simulink model "Power_System_33Bus_Modeling_test"  (R2024a)
settings: Solver=FixedStepAuto  StartTime=0.0  StopTime=0.2  RelTol=1e-3
libraries: spsThreePhaseSeriesRLCLoadLib x64, spsThreePhaseVIMeasurementLib x33, spsThreePhaseSeriesRLCBranchLib x32, spsRMSLib x2, spsThreePhaseSourceLib x1, spspowerguiLib x1
(part 2 of 2)

== system Power_System_33Bus_Modeling_test/Bus_21 ==
  Bus Load 21 : spsThreePhaseSeriesRLCLoadLib/Three-Phase Series RLC Load  LConnTagsString=A|B|C  Configuration=Y (grounded)  NominalVoltage=22900  Vabc=[1e3 1e3 1e3]  Vabcp=[1e3 1e3 1e3]  NominalFrequency=60  UnbalancedPower=off  ActivePower=450e3  InductivePower=200e3  CapacitivePower=0  Pabc=[10e3 9e3 11e3]  QLabc=[100 90 110]  QCabc=[100 90 110]  Pabcp=[10e3 9e3 11e3]  QLabcp=[100 90 110]  QCabcp=[100 90 110]  Measurements=None  LoadType=constant PQ
  Bus_21 : spsThreePhaseVIMeasurementLib/Three-Phase V-I Measurement  VoltageMeasurement=phase-to-phase  SetLabelV=off  LabelV=Vabc  Vpu=off  VpuLL=off  CurrentMeasurement=yes  SetLabelI=off  LabelI=Iabc  Ipu=off  Pbase=100e6  Vbase=500e3  OutputType=Complex  PhasorSimulation=off  PSBequivalent=0
  Capacitor 21 : spsThreePhaseSeriesRLCLoadLib/Three-Phase Series RLC Load  LConnTagsString=A|B|C  Configuration=Y (grounded)  NominalVoltage=22900  Vabc=[1e3 1e3 1e3]  Vabcp=[1e3 1e3 1e3]  NominalFrequency=60  UnbalancedPower=off  ActivePower=0  InductivePower=0  CapacitivePower=1e-06  Pabc=[10e3 9e3 11e3]  QLabc=[100 90 110]  QCabc=[100 90 110]  Pabcp=[10e3 9e3 11e3]  QLabcp=[100 90 110]  QCabcp=[100 90 110]  Measurements=None  LoadType=constant PQ
  VI Recorder2 : Subsystem
  InPhaseA : PMIOPort  Side=Left
  InPhaseB : PMIOPort  Port=2  Side=Left
  InPhaseC : PMIOPort  Port=3  Side=Left
  OutPhaseA : PMIOPort  Port=4  Side=Right
  OutPhaseB : PMIOPort  Port=5  Side=Right
  OutPhaseC : PMIOPort  Port=6  Side=Right
  wires:
  Bus_21/2 -> VI Recorder2/2(Irec)
  Bus_21/1 -> VI Recorder2/1(Vrec)
  connections:
  Bus Load 21/LConn1 -- Bus_21/RConn1 -- OutPhaseA/RConn1 -- Capacitor 21/LConn1
  Bus Load 21/LConn2 -- Bus_21/RConn2 -- Capacitor 21/LConn2 -- OutPhaseB/RConn1
  Bus_21/RConn3 -- Bus Load 21/LConn3 -- OutPhaseC/RConn1 -- Capacitor 21/LConn3
  InPhaseA/RConn1 -- Bus_21/LConn1
  Bus_21/LConn2 -- InPhaseB/RConn1
  InPhaseC/RConn1 -- Bus_21/LConn3

== system Power_System_33Bus_Modeling_test/Bus_22 ==
  Bus Load 22 : spsThreePhaseSeriesRLCLoadLib/Three-Phase Series RLC Load  LConnTagsString=A|B|C  Configuration=Y (grounded)  NominalVoltage=22900  Vabc=[1e3 1e3 1e3]  Vabcp=[1e3 1e3 1e3]  NominalFrequency=60  UnbalancedPower=off  ActivePower=450e3  InductivePower=200e3  CapacitivePower=0  Pabc=[10e3 9e3 11e3]  QLabc=[100 90 110]  QCabc=[100 90 110]  Pabcp=[10e3 9e3 11e3]  QLabcp=[100 90 110]  QCabcp=[100 90 110]  Measurements=None  LoadType=constant PQ
  Bus_22 : spsThreePhaseVIMeasurementLib/Three-Phase V-I Measurement  VoltageMeasurement=phase-to-phase  SetLabelV=off  LabelV=Vabc  Vpu=off  VpuLL=off  CurrentMeasurement=yes  SetLabelI=off  LabelI=Iabc  Ipu=off  Pbase=100e6  Vbase=500e3  OutputType=Complex  PhasorSimulation=off  PSBequivalent=0
  Capacitor 22 : spsThreePhaseSeriesRLCLoadLib/Three-Phase Series RLC Load  LConnTagsString=A|B|C  Configuration=Y (grounded)  NominalVoltage=22900  Vabc=[1e3 1e3 1e3]  Vabcp=[1e3 1e3 1e3]  NominalFrequency=60  UnbalancedPower=off  ActivePower=0  InductivePower=0  CapacitivePower=1e-06  Pabc=[10e3 9e3 11e3]  QLabc=[100 90 110]  QCabc=[100 90 110]  Pabcp=[10e3 9e3 11e3]  QLabcp=[100 90 110]  QCabcp=[100 90 110]  Measurements=None  LoadType=constant PQ
  VI Recorder3 : Subsystem
  InPhaseA : PMIOPort  Side=Left
  InPhaseB : PMIOPort  Port=2  Side=Left
  InPhaseC : PMIOPort  Port=3  Side=Left
  wires:
  Bus_22/2 -> VI Recorder3/2(Irec)
  Bus_22/1 -> VI Recorder3/1(Vrec)
  connections:
  Bus_22/RConn2 -- Capacitor 22/LConn2 -- Bus Load 22/LConn2
  Bus Load 22/LConn3 -- Capacitor 22/LConn3 -- Bus_22/RConn3
  Bus_22/RConn1 -- Capacitor 22/LConn1 -- Bus Load 22/LConn1
  InPhaseA/RConn1 -- Bus_22/LConn1
  InPhaseB/RConn1 -- Bus_22/LConn2
  InPhaseC/RConn1 -- Bus_22/LConn3

== system Power_System_33Bus_Modeling_test/Bus_23 ==
  Bus Load 23 : spsThreePhaseSeriesRLCLoadLib/Three-Phase Series RLC Load  LConnTagsString=A|B|C  Configuration=Y (grounded)  NominalVoltage=22900  Vabc=[1e3 1e3 1e3]  Vabcp=[1e3 1e3 1e3]  NominalFrequency=60  UnbalancedPower=off  ActivePower=450e3  InductivePower=250e3  CapacitivePower=0  Pabc=[10e3 9e3 11e3]  QLabc=[100 90 110]  QCabc=[100 90 110]  Pabcp=[10e3 9e3 11e3]  QLabcp=[100 90 110]  QCabcp=[100 90 110]  Measurements=None  LoadType=constant PQ
  Bus_23 : spsThreePhaseVIMeasurementLib/Three-Phase V-I Measurement  VoltageMeasurement=phase-to-phase  SetLabelV=off  LabelV=Vabc  Vpu=off  VpuLL=off  CurrentMeasurement=yes  SetLabelI=off  LabelI=Iabc  Ipu=off  Pbase=100e6  Vbase=500e3  OutputType=Complex  PhasorSimulation=off  PSBequivalent=0
  Capacitor 23 : spsThreePhaseSeriesRLCLoadLib/Three-Phase Series RLC Load  LConnTagsString=A|B|C  Configuration=Y (grounded)  NominalVoltage=22900  Vabc=[1e3 1e3 1e3]  Vabcp=[1e3 1e3 1e3]  NominalFrequency=60  UnbalancedPower=off  ActivePower=0  InductivePower=0  CapacitivePower=1e-06  Pabc=[10e3 9e3 11e3]  QLabc=[100 90 110]  QCabc=[100 90 110]  Pabcp=[10e3 9e3 11e3]  QLabcp=[100 90 110]  QCabcp=[100 90 110]  Measurements=None  LoadType=constant PQ
  VI Recorder32 : Subsystem
  InPhaseA : PMIOPort  Side=Left
  InPhaseB : PMIOPort  Port=2  Side=Left
  InPhaseC : PMIOPort  Port=3  Side=Left
  OutPhaseA : PMIOPort  Port=4  Side=Right
  OutPhaseB : PMIOPort  Port=5  Side=Right
  OutPhaseC : PMIOPort  Port=6  Side=Right
  wires:
  Bus_23/2 -> VI Recorder32/2(Irec)
  Bus_23/1 -> VI Recorder32/1(Vrec)
  connections:
  Bus_23/RConn1 -- OutPhaseA/RConn1 -- Capacitor 23/LConn1 -- Bus Load 23/LConn1
  Bus Load 23/LConn2 -- OutPhaseB/RConn1 -- Capacitor 23/LConn2 -- Bus_23/RConn2
  Bus Load 23/LConn3 -- OutPhaseC/RConn1 -- Capacitor 23/LConn3 -- Bus_23/RConn3
  InPhaseA/RConn1 -- Bus_23/LConn1
  InPhaseB/RConn1 -- Bus_23/LConn2
  InPhaseC/RConn1 -- Bus_23/LConn3

== system Power_System_33Bus_Modeling_test/Bus_24 ==
  Bus Load 24 : spsThreePhaseSeriesRLCLoadLib/Three-Phase Series RLC Load  LConnTagsString=A|B|C  Configuration=Y (grounded)  NominalVoltage=22900  Vabc=[1e3 1e3 1e3]  Vabcp=[1e3 1e3 1e3]  NominalFrequency=60  UnbalancedPower=off  ActivePower=2100e3  InductivePower=1000e3  CapacitivePower=0  Pabc=[10e3 9e3 11e3]  QLabc=[100 90 110]  QCabc=[100 90 110]  Pabcp=[10e3 9e3 11e3]  QLabcp=[100 90 110]  QCabcp=[100 90 110]  Measurements=None  LoadType=constant PQ
  Bus_24 : spsThreePhaseVIMeasurementLib/Three-Phase V-I Measurement  VoltageMeasurement=phase-to-phase  SetLabelV=off  LabelV=Vabc  Vpu=off  VpuLL=off  CurrentMeasurement=yes  SetLabelI=off  LabelI=Iabc  Ipu=off  Pbase=100e6  Vbase=500e3  OutputType=Complex  PhasorSimulation=off  PSBequivalent=0
  Capacitor 24 : spsThreePhaseSeriesRLCLoadLib/Three-Phase Series RLC Load  LConnTagsString=A|B|C  Configuration=Y (grounded)  NominalVoltage=22900  Vabc=[1e3 1e3 1e3]  Vabcp=[1e3 1e3 1e3]  NominalFrequency=60  UnbalancedPower=off  ActivePower=0  InductivePower=0  CapacitivePower=1e-06  Pabc=[10e3 9e3 11e3]  QLabc=[100 90 110]  QCabc=[100 90 110]  Pabcp=[10e3 9e3 11e3]  QLabcp=[100 90 110]  QCabcp=[100 90 110]  Measurements=None  LoadType=constant PQ
  VI Recorder31 : Subsystem
  InPhaseA : PMIOPort  Side=Left
  InPhaseB : PMIOPort  Port=2  Side=Left
  InPhaseC : PMIOPort  Port=3  Side=Left
  OutPhaseA : PMIOPort  Port=4  Side=Right
  OutPhaseB : PMIOPort  Port=5  Side=Right
  OutPhaseC : PMIOPort  Port=6  Side=Right
  wires:
  Bus_24/1 -> VI Recorder31/1(Vrec)
  Bus_24/2 -> VI Recorder31/2(Irec)
  connections:
  Bus_24/RConn1 -- OutPhaseA/RConn1 -- Capacitor 24/LConn1 -- Bus Load 24/LConn1
  Bus Load 24/LConn2 -- OutPhaseB/RConn1 -- Capacitor 24/LConn2 -- Bus_24/RConn2
  InPhaseA/RConn1 -- Bus_24/LConn1
  InPhaseB/RConn1 -- Bus_24/LConn2
  InPhaseC/RConn1 -- Bus_24/LConn3
  Bus Load 24/LConn3 -- OutPhaseC/RConn1 -- Capacitor 24/LConn3 -- Bus_24/RConn3

== system Power_System_33Bus_Modeling_test/Bus_25 ==
  Bus Load 25 : spsThreePhaseSeriesRLCLoadLib/Three-Phase Series RLC Load  LConnTagsString=A|B|C  Configuration=Y (grounded)  NominalVoltage=22900  Vabc=[1e3 1e3 1e3]  Vabcp=[1e3 1e3 1e3]  NominalFrequency=60  UnbalancedPower=off  ActivePower=2100e3  InductivePower=1000e3  CapacitivePower=0  Pabc=[10e3 9e3 11e3]  QLabc=[100 90 110]  QCabc=[100 90 110]  Pabcp=[10e3 9e3 11e3]  QLabcp=[100 90 110]  QCabcp=[100 90 110]  Measurements=None  LoadType=constant PQ
  Bus_25 : spsThreePhaseVIMeasurementLib/Three-Phase V-I Measurement  VoltageMeasurement=phase-to-phase  SetLabelV=off  LabelV=Vabc  Vpu=off  VpuLL=off  CurrentMeasurement=yes  SetLabelI=off  LabelI=Iabc  Ipu=off  Pbase=100e6  Vbase=500e3  OutputType=Complex  PhasorSimulation=off  PSBequivalent=0
  Capacitor 25 : spsThreePhaseSeriesRLCLoadLib/Three-Phase Series RLC Load  LConnTagsString=A|B|C  Configuration=Y (grounded)  NominalVoltage=22900  Vabc=[1e3 1e3 1e3]  Vabcp=[1e3 1e3 1e3]  NominalFrequency=60  UnbalancedPower=off  ActivePower=0  InductivePower=0  CapacitivePower=1e-06  Pabc=[10e3 9e3 11e3]  QLabc=[100 90 110]  QCabc=[100 90 110]  Pabcp=[10e3 9e3 11e3]  QLabcp=[100 90 110]  QCabcp=[100 90 110]  Measurements=None  LoadType=constant PQ
  VI Recorder30 : Subsystem
  InPhaseA : PMIOPort  Side=Left
  InPhaseB : PMIOPort  Port=2  Side=Left
  InPhaseC : PMIOPort  Port=3  Side=Left
  wires:
  Bus_25/2 -> VI Recorder30/2(Irec)
  Bus_25/1 -> VI Recorder30/1(Vrec)
  connections:
  Bus Load 25/LConn1 -- Capacitor 25/LConn1 -- Bus_25/RConn1
  Bus_25/RConn2 -- Capacitor 25/LConn2 -- Bus Load 25/LConn2
  Bus Load 25/LConn3 -- Capacitor 25/LConn3 -- Bus_25/RConn3
  InPhaseB/RConn1 -- Bus_25/LConn2
  InPhaseA/RConn1 -- Bus_25/LConn1
  InPhaseC/RConn1 -- Bus_25/LConn3

== system Power_System_33Bus_Modeling_test/Bus_26 ==
  Bus Load 26 : spsThreePhaseSeriesRLCLoadLib/Three-Phase Series RLC Load  LConnTagsString=A|B|C  Configuration=Y (grounded)  NominalVoltage=22900  Vabc=[1e3 1e3 1e3]  Vabcp=[1e3 1e3 1e3]  NominalFrequency=60  UnbalancedPower=off  ActivePower=300e3  InductivePower=125e3  CapacitivePower=0  Pabc=[10e3 9e3 11e3]  QLabc=[100 90 110]  QCabc=[100 90 110]  Pabcp=[10e3 9e3 11e3]  QLabcp=[100 90 110]  QCabcp=[100 90 110]  Measurements=None  LoadType=constant PQ
  Bus_26 : spsThreePhaseVIMeasurementLib/Three-Phase V-I Measurement  VoltageMeasurement=phase-to-phase  SetLabelV=off  LabelV=Vabc  Vpu=off  VpuLL=off  CurrentMeasurement=yes  SetLabelI=off  LabelI=Iabc  Ipu=off  Pbase=100e6  Vbase=500e3  OutputType=Complex  PhasorSimulation=off  PSBequivalent=0
  Capacitor 26 : spsThreePhaseSeriesRLCLoadLib/Three-Phase Series RLC Load  LConnTagsString=A|B|C  Configuration=Y (grounded)  NominalVoltage=22900  Vabc=[1e3 1e3 1e3]  Vabcp=[1e3 1e3 1e3]  NominalFrequency=60  UnbalancedPower=off  ActivePower=0  InductivePower=0  CapacitivePower=1e-06  Pabc=[10e3 9e3 11e3]  QLabc=[100 90 110]  QCabc=[100 90 110]  Pabcp=[10e3 9e3 11e3]  QLabcp=[100 90 110]  QCabcp=[100 90 110]  Measurements=None  LoadType=constant PQ
  VI Recorder22 : Subsystem
  InPhaseA : PMIOPort  Side=Left
  InPhaseB : PMIOPort  Port=2  Side=Left
  InPhaseC : PMIOPort  Port=3  Side=Left
  OutPhaseA : PMIOPort  Port=4  Side=Right
  OutPhaseB : PMIOPort  Port=5  Side=Right
  OutPhaseC : PMIOPort  Port=6  Side=Right
  wires:
  Bus_26/2 -> VI Recorder22/2(Irec)
  Bus_26/1 -> VI Recorder22/1(Vrec)
  connections:
  Bus_26/RConn3 -- OutPhaseC/RConn1 -- Capacitor 26/LConn3 -- Bus Load 26/LConn3
  Bus Load 26/LConn2 -- OutPhaseB/RConn1 -- Capacitor 26/LConn2 -- Bus_26/RConn2
  Bus_26/RConn1 -- OutPhaseA/RConn1 -- Capacitor 26/LConn1 -- Bus Load 26/LConn1
  InPhaseA/RConn1 -- Bus_26/LConn1
  InPhaseB/RConn1 -- Bus_26/LConn2
  InPhaseC/RConn1 -- Bus_26/LConn3

== system Power_System_33Bus_Modeling_test/Bus_27 ==
  Bus Load 27 : spsThreePhaseSeriesRLCLoadLib/Three-Phase Series RLC Load  LConnTagsString=A|B|C  Configuration=Y (grounded)  NominalVoltage=22900  Vabc=[1e3 1e3 1e3]  Vabcp=[1e3 1e3 1e3]  NominalFrequency=60  UnbalancedPower=off  ActivePower=300e3  InductivePower=125e3  CapacitivePower=0  Pabc=[10e3 9e3 11e3]  QLabc=[100 90 110]  QCabc=[100 90 110]  Pabcp=[10e3 9e3 11e3]  QLabcp=[100 90 110]  QCabcp=[100 90 110]  Measurements=None  LoadType=constant PQ
  Bus_27 : spsThreePhaseVIMeasurementLib/Three-Phase V-I Measurement  VoltageMeasurement=phase-to-phase  SetLabelV=off  LabelV=Vabc  Vpu=off  VpuLL=off  CurrentMeasurement=yes  SetLabelI=off  LabelI=Iabc  Ipu=off  Pbase=100e6  Vbase=500e3  OutputType=Complex  PhasorSimulation=off  PSBequivalent=0
  Capacitor 27 : spsThreePhaseSeriesRLCLoadLib/Three-Phase Series RLC Load  LConnTagsString=A|B|C  Configuration=Y (grounded)  NominalVoltage=22900  Vabc=[1e3 1e3 1e3]  Vabcp=[1e3 1e3 1e3]  NominalFrequency=60  UnbalancedPower=off  ActivePower=0  InductivePower=0  CapacitivePower=1e-06  Pabc=[10e3 9e3 11e3]  QLabc=[100 90 110]  QCabc=[100 90 110]  Pabcp=[10e3 9e3 11e3]  QLabcp=[100 90 110]  QCabcp=[100 90 110]  Measurements=None  LoadType=constant PQ
  VI Recorder23 : Subsystem
  InPhaseA : PMIOPort  Side=Left
  InPhaseB : PMIOPort  Port=2  Side=Left
  InPhaseC : PMIOPort  Port=3  Side=Left
  OutPhaseA : PMIOPort  Port=4  Side=Right
  OutPhaseB : PMIOPort  Port=5  Side=Right
  OutPhaseC : PMIOPort  Port=6  Side=Right
  wires:
  Bus_27/1 -> VI Recorder23/1(Vrec)
  Bus_27/2 -> VI Recorder23/2(Irec)
  connections:
  Bus Load 27/LConn1 -- Bus_27/RConn1 -- OutPhaseA/RConn1 -- Capacitor 27/LConn1
  Bus Load 27/LConn2 -- Bus_27/RConn2 -- OutPhaseB/RConn1 -- Capacitor 27/LConn2
  Bus_27/RConn3 -- OutPhaseC/RConn1 -- Capacitor 27/LConn3 -- Bus Load 27/LConn3
  InPhaseA/RConn1 -- Bus_27/LConn1
  InPhaseB/RConn1 -- Bus_27/LConn2
  InPhaseC/RConn1 -- Bus_27/LConn3

== system Power_System_33Bus_Modeling_test/Bus_28 ==
  Bus Load 28 : spsThreePhaseSeriesRLCLoadLib/Three-Phase Series RLC Load  LConnTagsString=A|B|C  Configuration=Y (grounded)  NominalVoltage=22900  Vabc=[1e3 1e3 1e3]  Vabcp=[1e3 1e3 1e3]  NominalFrequency=60  UnbalancedPower=off  ActivePower=300e3  InductivePower=100e3  CapacitivePower=0  Pabc=[10e3 9e3 11e3]  QLabc=[100 90 110]  QCabc=[100 90 110]  Pabcp=[10e3 9e3 11e3]  QLabcp=[100 90 110]  QCabcp=[100 90 110]  Measurements=None  LoadType=constant PQ
  Bus_28 : spsThreePhaseVIMeasurementLib/Three-Phase V-I Measurement  VoltageMeasurement=phase-to-phase  SetLabelV=off  LabelV=Vabc  Vpu=off  VpuLL=off  CurrentMeasurement=yes  SetLabelI=off  LabelI=Iabc  Ipu=off  Pbase=100e6  Vbase=500e3  OutputType=Complex  PhasorSimulation=off  PSBequivalent=0
  Capacitor 28 : spsThreePhaseSeriesRLCLoadLib/Three-Phase Series RLC Load  LConnTagsString=A|B|C  Configuration=Y (grounded)  NominalVoltage=22900  Vabc=[1e3 1e3 1e3]  Vabcp=[1e3 1e3 1e3]  NominalFrequency=60  UnbalancedPower=off  ActivePower=0  InductivePower=0  CapacitivePower=1e-06  Pabc=[10e3 9e3 11e3]  QLabc=[100 90 110]  QCabc=[100 90 110]  Pabcp=[10e3 9e3 11e3]  QLabcp=[100 90 110]  QCabcp=[100 90 110]  Measurements=None  LoadType=constant PQ
  VI Recorder24 : Subsystem
  InPhaseA : PMIOPort  Side=Left
  InPhaseB : PMIOPort  Port=2  Side=Left
  InPhaseC : PMIOPort  Port=3  Side=Left
  OutPhaseA : PMIOPort  Port=4  Side=Right
  OutPhaseB : PMIOPort  Port=5  Side=Right
  OutPhaseC : PMIOPort  Port=6  Side=Right
  wires:
  Bus_28/2 -> VI Recorder24/2(Irec)
  Bus_28/1 -> VI Recorder24/1(Vrec)
  connections:
  Bus Load 28/LConn1 -- OutPhaseA/RConn1 -- Capacitor 28/LConn1 -- Bus_28/RConn1
  Bus Load 28/LConn2 -- OutPhaseB/RConn1 -- Capacitor 28/LConn2 -- Bus_28/RConn2
  Bus Load 28/LConn3 -- OutPhaseC/RConn1 -- Capacitor 28/LConn3 -- Bus_28/RConn3
  InPhaseA/RConn1 -- Bus_28/LConn1
  InPhaseB/RConn1 -- Bus_28/LConn2
  InPhaseC/RConn1 -- Bus_28/LConn3

== system Power_System_33Bus_Modeling_test/Bus_29 ==
  Bus Load 29 : spsThreePhaseSeriesRLCLoadLib/Three-Phase Series RLC Load  LConnTagsString=A|B|C  Configuration=Y (grounded)  NominalVoltage=22900  Vabc=[1e3 1e3 1e3]  Vabcp=[1e3 1e3 1e3]  NominalFrequency=60  UnbalancedPower=off  ActivePower=600e3  InductivePower=350e3  CapacitivePower=0  Pabc=[10e3 9e3 11e3]  QLabc=[100 90 110]  QCabc=[100 90 110]  Pabcp=[10e3 9e3 11e3]  QLabcp=[100 90 110]  QCabcp=[100 90 110]  Measurements=None  LoadType=constant PQ
  Bus_29 : spsThreePhaseVIMeasurementLib/Three-Phase V-I Measurement  VoltageMeasurement=phase-to-phase  SetLabelV=off  LabelV=Vabc  Vpu=off  VpuLL=off  CurrentMeasurement=yes  SetLabelI=off  LabelI=Iabc  Ipu=off  Pbase=100e6  Vbase=500e3  OutputType=Complex  PhasorSimulation=off  PSBequivalent=0
  Capacitor 29 : spsThreePhaseSeriesRLCLoadLib/Three-Phase Series RLC Load  LConnTagsString=A|B|C  Configuration=Y (grounded)  NominalVoltage=22900  Vabc=[1e3 1e3 1e3]  Vabcp=[1e3 1e3 1e3]  NominalFrequency=60  UnbalancedPower=off  ActivePower=0  InductivePower=0  CapacitivePower=1e-06  Pabc=[10e3 9e3 11e3]  QLabc=[100 90 110]  QCabc=[100 90 110]  Pabcp=[10e3 9e3 11e3]  QLabcp=[100 90 110]  QCabcp=[100 90 110]  Measurements=None  LoadType=constant PQ
  VI Recorder25 : Subsystem
  InPhaseA : PMIOPort  Side=Left
  InPhaseB : PMIOPort  Port=2  Side=Left
  InPhaseC : PMIOPort  Port=3  Side=Left
  OutPhaseA : PMIOPort  Port=4  Side=Right
  OutPhaseB : PMIOPort  Port=5  Side=Right
  OutPhaseC : PMIOPort  Port=6  Side=Right
  wires:
  Bus_29/1 -> VI Recorder25/1(Vrec)
  Bus_29/2 -> VI Recorder25/2(Irec)
  connections:
  Bus_29/RConn1 -- OutPhaseA/RConn1 -- Capacitor 29/LConn1 -- Bus Load 29/LConn1
  Bus Load 29/LConn2 -- OutPhaseB/RConn1 -- Capacitor 29/LConn2 -- Bus_29/RConn2
  Bus Load 29/LConn3 -- OutPhaseC/RConn1 -- Capacitor 29/LConn3 -- Bus_29/RConn3
  InPhaseB/RConn1 -- Bus_29/LConn2
  InPhaseA/RConn1 -- Bus_29/LConn1
  InPhaseC/RConn1 -- Bus_29/LConn3

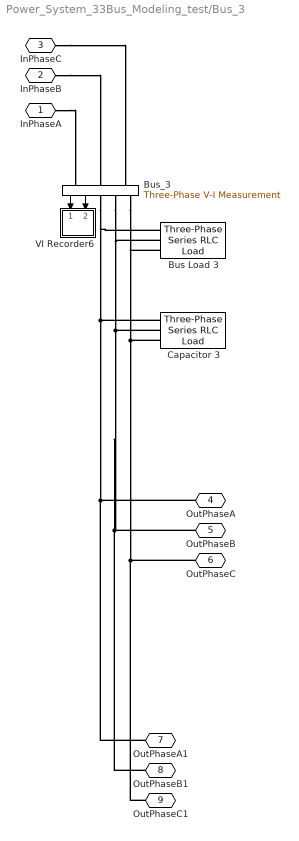
== system Power_System_33Bus_Modeling_test/Bus_3 ==
  Bus Load 3 : spsThreePhaseSeriesRLCLoadLib/Three-Phase Series RLC Load  LConnTagsString=A|B|C  Configuration=Y (grounded)  NominalVoltage=22900  Vabc=[1e3 1e3 1e3]  Vabcp=[1e3 1e3 1e3]  NominalFrequency=60  UnbalancedPower=off  ActivePower=450e3  InductivePower=200e3  CapacitivePower=0  Pabc=[10e3 9e3 11e3]  QLabc=[100 90 110]  QCabc=[100 90 110]  Pabcp=[10e3 9e3 11e3]  QLabcp=[100 90 110]  QCabcp=[100 90 110]  Measurements=None  LoadType=constant PQ
  Bus_3 : spsThreePhaseVIMeasurementLib/Three-Phase V-I Measurement  VoltageMeasurement=phase-to-phase  SetLabelV=off  LabelV=Vabc  Vpu=off  VpuLL=off  CurrentMeasurement=yes  SetLabelI=off  LabelI=Iabc  Ipu=off  Pbase=100e6  Vbase=500e3  OutputType=Complex  PhasorSimulation=off  PSBequivalent=0
  Capacitor 3 : spsThreePhaseSeriesRLCLoadLib/Three-Phase Series RLC Load  LConnTagsString=A|B|C  Configuration=Y (grounded)  NominalVoltage=22900  Vabc=[1e3 1e3 1e3]  Vabcp=[1e3 1e3 1e3]  NominalFrequency=60  UnbalancedPower=off  ActivePower=0  InductivePower=0  CapacitivePower=1e-06  Pabc=[10e3 9e3 11e3]  QLabc=[100 90 110]  QCabc=[100 90 110]  Pabcp=[10e3 9e3 11e3]  QLabcp=[100 90 110]  QCabcp=[100 90 110]  Measurements=None  LoadType=constant PQ
  VI Recorder6 : Subsystem
  InPhaseA : PMIOPort  Side=Left
  InPhaseB : PMIOPort  Port=2  Side=Left
  InPhaseC : PMIOPort  Port=3  Side=Left
  OutPhaseA : PMIOPort  Port=4  Side=Right
  OutPhaseB : PMIOPort  Port=5  Side=Right
  OutPhaseC : PMIOPort  Port=6  Side=Right
  OutPhaseA1 : PMIOPort  Port=7  Side=Right
  OutPhaseB1 : PMIOPort  Port=8  Side=Right
  OutPhaseC1 : PMIOPort  Port=9  Side=Right
  wires:
  Bus_3/2 -> VI Recorder6/2(Irec)
  Bus_3/1 -> VI Recorder6/1(Vrec)
  connections:
  Capacitor 3/LConn1 -- Bus Load 3/LConn1 -- Bus_3/RConn1 -- OutPhaseA1/RConn1 -- OutPhaseA/RConn1
  Capacitor 3/LConn2 -- Bus Load 3/LConn2 -- Bus_3/RConn2 -- OutPhaseB1/RConn1 -- OutPhaseB/RConn1
  Capacitor 3/LConn3 -- Bus_3/RConn3 -- Bus Load 3/LConn3 -- OutPhaseC1/RConn1 -- OutPhaseC/RConn1
  InPhaseA/RConn1 -- Bus_3/LConn1
  InPhaseB/RConn1 -- Bus_3/LConn2
  InPhaseC/RConn1 -- Bus_3/LConn3

== system Power_System_33Bus_Modeling_test/Bus_30 ==
  Bus Load 30 : spsThreePhaseSeriesRLCLoadLib/Three-Phase Series RLC Load  LConnTagsString=A|B|C  Configuration=Y (grounded)  NominalVoltage=22900  Vabc=[1e3 1e3 1e3]  Vabcp=[1e3 1e3 1e3]  NominalFrequency=60  UnbalancedPower=off  ActivePower=1000e3  InductivePower=3000e3  CapacitivePower=0  Pabc=[10e3 9e3 11e3]  QLabc=[100 90 110]  QCabc=[100 90 110]  Pabcp=[10e3 9e3 11e3]  QLabcp=[100 90 110]  QCabcp=[100 90 110]  Measurements=None  LoadType=constant PQ
  Bus_30 : spsThreePhaseVIMeasurementLib/Three-Phase V-I Measurement  VoltageMeasurement=phase-to-phase  SetLabelV=off  LabelV=Vabc  Vpu=off  VpuLL=off  CurrentMeasurement=yes  SetLabelI=off  LabelI=Iabc  Ipu=off  Pbase=100e6  Vbase=500e3  OutputType=Complex  PhasorSimulation=off  PSBequivalent=0
  Capacitor 30 : spsThreePhaseSeriesRLCLoadLib/Three-Phase Series RLC Load  LConnTagsString=A|B|C  Configuration=Y (grounded)  NominalVoltage=22900  Vabc=[1e3 1e3 1e3]  Vabcp=[1e3 1e3 1e3]  NominalFrequency=60  UnbalancedPower=off  ActivePower=0  InductivePower=0  CapacitivePower=1e-06  Pabc=[10e3 9e3 11e3]  QLabc=[100 90 110]  QCabc=[100 90 110]  Pabcp=[10e3 9e3 11e3]  QLabcp=[100 90 110]  QCabcp=[100 90 110]  Measurements=None  LoadType=constant PQ
  VI Recorder26 : Subsystem
  InPhaseA : PMIOPort  Side=Left
  InPhaseB : PMIOPort  Port=2  Side=Left
  InPhaseC : PMIOPort  Port=3  Side=Left
  OutPhaseA : PMIOPort  Port=4  Side=Right
  OutPhaseB : PMIOPort  Port=5  Side=Right
  OutPhaseC : PMIOPort  Port=6  Side=Right
  wires:
  Bus_30/1 -> VI Recorder26/1(Vrec)
  Bus_30/2 -> VI Recorder26/2(Irec)
  connections:
  Bus_30/RConn1 -- OutPhaseA/RConn1 -- Capacitor 30/LConn1 -- Bus Load 30/LConn1
  Bus Load 30/LConn2 -- OutPhaseB/RConn1 -- Capacitor 30/LConn2 -- Bus_30/RConn2
  Bus Load 30/LConn3 -- OutPhaseC/RConn1 -- Capacitor 30/LConn3 -- Bus_30/RConn3
  InPhaseB/RConn1 -- Bus_30/LConn2
  InPhaseA/RConn1 -- Bus_30/LConn1
  InPhaseC/RConn1 -- Bus_30/LConn3

== system Power_System_33Bus_Modeling_test/Bus_31 ==
  Bus Load 31 : spsThreePhaseSeriesRLCLoadLib/Three-Phase Series RLC Load  LConnTagsString=A|B|C  Configuration=Y (grounded)  NominalVoltage=22900  Vabc=[1e3 1e3 1e3]  Vabcp=[1e3 1e3 1e3]  NominalFrequency=60  UnbalancedPower=off  ActivePower=750e3  InductivePower=350e3  CapacitivePower=0  Pabc=[10e3 9e3 11e3]  QLabc=[100 90 110]  QCabc=[100 90 110]  Pabcp=[10e3 9e3 11e3]  QLabcp=[100 90 110]  QCabcp=[100 90 110]  Measurements=None  LoadType=constant PQ
  Bus_31 : spsThreePhaseVIMeasurementLib/Three-Phase V-I Measurement  VoltageMeasurement=phase-to-phase  SetLabelV=off  LabelV=Vabc  Vpu=off  VpuLL=off  CurrentMeasurement=yes  SetLabelI=off  LabelI=Iabc  Ipu=off  Pbase=100e6  Vbase=500e3  OutputType=Complex  PhasorSimulation=off  PSBequivalent=0
  Capacitor 31 : spsThreePhaseSeriesRLCLoadLib/Three-Phase Series RLC Load  LConnTagsString=A|B|C  Configuration=Y (grounded)  NominalVoltage=22900  Vabc=[1e3 1e3 1e3]  Vabcp=[1e3 1e3 1e3]  NominalFrequency=60  UnbalancedPower=off  ActivePower=0  InductivePower=0  CapacitivePower=1e-06  Pabc=[10e3 9e3 11e3]  QLabc=[100 90 110]  QCabc=[100 90 110]  Pabcp=[10e3 9e3 11e3]  QLabcp=[100 90 110]  QCabcp=[100 90 110]  Measurements=None  LoadType=constant PQ
  VI Recorder27 : Subsystem
  InPhaseA : PMIOPort  Side=Left
  InPhaseB : PMIOPort  Port=2  Side=Left
  InPhaseC : PMIOPort  Port=3  Side=Left
  OutPhaseA : PMIOPort  Port=4  Side=Right
  OutPhaseB : PMIOPort  Port=5  Side=Right
  OutPhaseC : PMIOPort  Port=6  Side=Right
  wires:
  Bus_31/2 -> VI Recorder27/2(Irec)
  Bus_31/1 -> VI Recorder27/1(Vrec)
  connections:
  Bus_31/RConn1 -- OutPhaseA/RConn1 -- Capacitor 31/LConn1 -- Bus Load 31/LConn1
  Bus Load 31/LConn2 -- OutPhaseB/RConn1 -- Capacitor 31/LConn2 -- Bus_31/RConn2
  Bus Load 31/LConn3 -- OutPhaseC/RConn1 -- Capacitor 31/LConn3 -- Bus_31/RConn3
  InPhaseA/RConn1 -- Bus_31/LConn1
  Bus_31/LConn2 -- InPhaseB/RConn1
  InPhaseC/RConn1 -- Bus_31/LConn3

== system Power_System_33Bus_Modeling_test/Bus_32 ==
  Bus Load 32 : spsThreePhaseSeriesRLCLoadLib/Three-Phase Series RLC Load  LConnTagsString=A|B|C  Configuration=Y (grounded)  NominalVoltage=22900  Vabc=[1e3 1e3 1e3]  Vabcp=[1e3 1e3 1e3]  NominalFrequency=60  UnbalancedPower=off  ActivePower=1050e3  InductivePower=500e3  CapacitivePower=0  Pabc=[10e3 9e3 11e3]  QLabc=[100 90 110]  QCabc=[100 90 110]  Pabcp=[10e3 9e3 11e3]  QLabcp=[100 90 110]  QCabcp=[100 90 110]  Measurements=None  LoadType=constant PQ
  Bus_32 : spsThreePhaseVIMeasurementLib/Three-Phase V-I Measurement  VoltageMeasurement=phase-to-phase  SetLabelV=off  LabelV=Vabc  Vpu=off  VpuLL=off  CurrentMeasurement=yes  SetLabelI=off  LabelI=Iabc  Ipu=off  Pbase=100e6  Vbase=500e3  OutputType=Complex  PhasorSimulation=off  PSBequivalent=0
  Capacitor 32 : spsThreePhaseSeriesRLCLoadLib/Three-Phase Series RLC Load  LConnTagsString=A|B|C  Configuration=Y (grounded)  NominalVoltage=22900  Vabc=[1e3 1e3 1e3]  Vabcp=[1e3 1e3 1e3]  NominalFrequency=60  UnbalancedPower=off  ActivePower=0  InductivePower=0  CapacitivePower=1e-06  Pabc=[10e3 9e3 11e3]  QLabc=[100 90 110]  QCabc=[100 90 110]  Pabcp=[10e3 9e3 11e3]  QLabcp=[100 90 110]  QCabcp=[100 90 110]  Measurements=None  LoadType=constant PQ
  VI Recorder28 : Subsystem
  InPhaseA : PMIOPort  Side=Left
  InPhaseB : PMIOPort  Port=2  Side=Left
  InPhaseC : PMIOPort  Port=3  Side=Left
  OutPhaseA : PMIOPort  Port=4  Side=Right
  OutPhaseB : PMIOPort  Port=5  Side=Right
  OutPhaseC : PMIOPort  Port=6  Side=Right
  wires:
  Bus_32/2 -> VI Recorder28/2(Irec)
  Bus_32/1 -> VI Recorder28/1(Vrec)
  connections:
  Bus_32/RConn1 -- OutPhaseA/RConn1 -- Capacitor 32/LConn1 -- Bus Load 32/LConn1
  Bus_32/RConn3 -- OutPhaseC/RConn1 -- Capacitor 32/LConn3 -- Bus Load 32/LConn3
  Bus Load 32/LConn2 -- OutPhaseB/RConn1 -- Capacitor 32/LConn2 -- Bus_32/RConn2
  InPhaseA/RConn1 -- Bus_32/LConn1
  InPhaseB/RConn1 -- Bus_32/LConn2
  InPhaseC/RConn1 -- Bus_32/LConn3

== system Power_System_33Bus_Modeling_test/Bus_33 ==
  Bus Load 33 : spsThreePhaseSeriesRLCLoadLib/Three-Phase Series RLC Load  LConnTagsString=A|B|C  Configuration=Y (grounded)  NominalVoltage=22900  Vabc=[1e3 1e3 1e3]  Vabcp=[1e3 1e3 1e3]  NominalFrequency=60  UnbalancedPower=off  ActivePower=300e3  InductivePower=200e3  CapacitivePower=0  Pabc=[10e3 9e3 11e3]  QLabc=[100 90 110]  QCabc=[100 90 110]  Pabcp=[10e3 9e3 11e3]  QLabcp=[100 90 110]  QCabcp=[100 90 110]  Measurements=None  LoadType=constant PQ
  Bus_33 : spsThreePhaseVIMeasurementLib/Three-Phase V-I Measurement  VoltageMeasurement=phase-to-phase  SetLabelV=off  LabelV=Vabc  Vpu=off  VpuLL=off  CurrentMeasurement=yes  SetLabelI=off  LabelI=Iabc  Ipu=off  Pbase=100e6  Vbase=500e3  OutputType=Complex  PhasorSimulation=off  PSBequivalent=0
  Capacitor 33 : spsThreePhaseSeriesRLCLoadLib/Three-Phase Series RLC Load  LConnTagsString=A|B|C  Configuration=Y (grounded)  NominalVoltage=22900  Vabc=[1e3 1e3 1e3]  Vabcp=[1e3 1e3 1e3]  NominalFrequency=60  UnbalancedPower=off  ActivePower=0  InductivePower=0  CapacitivePower=1e-06  Pabc=[10e3 9e3 11e3]  QLabc=[100 90 110]  QCabc=[100 90 110]  Pabcp=[10e3 9e3 11e3]  QLabcp=[100 90 110]  QCabcp=[100 90 110]  Measurements=None  LoadType=constant PQ
  VI Recorder29 : Subsystem
  InPhaseA : PMIOPort  Side=Left
  InPhaseB : PMIOPort  Port=2  Side=Left
  InPhaseC : PMIOPort  Port=3  Side=Left
  wires:
  Bus_33/2 -> VI Recorder29/2(Irec)
  Bus_33/1 -> VI Recorder29/1(Vrec)
  connections:
  Bus Load 33/LConn1 -- Capacitor 33/LConn1 -- Bus_33/RConn1
  Bus Load 33/LConn2 -- Capacitor 33/LConn2 -- Bus_33/RConn2
  Bus_33/RConn3 -- Capacitor 33/LConn3 -- Bus Load 33/LConn3
  InPhaseA/RConn1 -- Bus_33/LConn1
  InPhaseB/RConn1 -- Bus_33/LConn2
  InPhaseC/RConn1 -- Bus_33/LConn3

== system Power_System_33Bus_Modeling_test/Bus_4 ==
  Bus Load 4 : spsThreePhaseSeriesRLCLoadLib/Three-Phase Series RLC Load  LConnTagsString=A|B|C  Configuration=Y (grounded)  NominalVoltage=22900  Vabc=[1e3 1e3 1e3]  Vabcp=[1e3 1e3 1e3]  NominalFrequency=60  UnbalancedPower=off  ActivePower=600e3  InductivePower=400e3  CapacitivePower=0  Pabc=[10e3 9e3 11e3]  QLabc=[100 90 110]  QCabc=[100 90 110]  Pabcp=[10e3 9e3 11e3]  QLabcp=[100 90 110]  QCabcp=[100 90 110]  Measurements=None  LoadType=constant PQ
  Bus_4 : spsThreePhaseVIMeasurementLib/Three-Phase V-I Measurement  VoltageMeasurement=phase-to-phase  SetLabelV=off  LabelV=Vabc  Vpu=off  VpuLL=off  CurrentMeasurement=yes  SetLabelI=off  LabelI=Iabc  Ipu=off  Pbase=100e6  Vbase=500e3  OutputType=Complex  PhasorSimulation=off  PSBequivalent=0
  Capacitor 4 : spsThreePhaseSeriesRLCLoadLib/Three-Phase Series RLC Load  LConnTagsString=A|B|C  Configuration=Y (grounded)  NominalVoltage=22900  Vabc=[1e3 1e3 1e3]  Vabcp=[1e3 1e3 1e3]  NominalFrequency=60  UnbalancedPower=off  ActivePower=0  InductivePower=0  CapacitivePower=1e-06  Pabc=[10e3 9e3 11e3]  QLabc=[100 90 110]  QCabc=[100 90 110]  Pabcp=[10e3 9e3 11e3]  QLabcp=[100 90 110]  QCabcp=[100 90 110]  Measurements=None  LoadType=constant PQ
  VI Recorder7 : Subsystem
  InPhaseA : PMIOPort  Side=Left
  InPhaseB : PMIOPort  Port=2  Side=Left
  InPhaseC : PMIOPort  Port=3  Side=Left
  OutPhaseA : PMIOPort  Port=4  Side=Right
  OutPhaseB : PMIOPort  Port=5  Side=Right
  OutPhaseC : PMIOPort  Port=6  Side=Right
  wires:
  Bus_4/1 -> VI Recorder7/1(Vrec)
  Bus_4/2 -> VI Recorder7/2(Irec)
  connections:
  Bus_4/RConn1 -- OutPhaseA/RConn1 -- Capacitor 4/LConn1 -- Bus Load 4/LConn1
  Bus Load 4/LConn2 -- OutPhaseB/RConn1 -- Capacitor 4/LConn2 -- Bus_4/RConn2
  Bus_4/RConn3 -- OutPhaseC/RConn1 -- Capacitor 4/LConn3 -- Bus Load 4/LConn3
  InPhaseA/RConn1 -- Bus_4/LConn1
  InPhaseB/RConn1 -- Bus_4/LConn2
  InPhaseC/RConn1 -- Bus_4/LConn3

== system Power_System_33Bus_Modeling_test/Bus_5 ==
  Bus Load 5 : spsThreePhaseSeriesRLCLoadLib/Three-Phase Series RLC Load  LConnTagsString=A|B|C  Configuration=Y (grounded)  NominalVoltage=22900  Vabc=[1e3 1e3 1e3]  Vabcp=[1e3 1e3 1e3]  NominalFrequency=50  UnbalancedPower=off  ActivePower=300e3  InductivePower=150e3  CapacitivePower=0  Pabc=[10e3 9e3 11e3]  QLabc=[100 90 110]  QCabc=[100 90 110]  Pabcp=[10e3 9e3 11e3]  QLabcp=[100 90 110]  QCabcp=[100 90 110]  Measurements=None  LoadType=constant PQ
  Bus_5 : spsThreePhaseVIMeasurementLib/Three-Phase V-I Measurement  VoltageMeasurement=phase-to-phase  SetLabelV=off  LabelV=Vabc  Vpu=off  VpuLL=off  CurrentMeasurement=yes  SetLabelI=off  LabelI=Iabc  Ipu=off  Pbase=100e6  Vbase=500e3  OutputType=Complex  PhasorSimulation=off  PSBequivalent=0
  Capacitor 5 : spsThreePhaseSeriesRLCLoadLib/Three-Phase Series RLC Load  LConnTagsString=A|B|C  Configuration=Y (grounded)  NominalVoltage=22900  Vabc=[1e3 1e3 1e3]  Vabcp=[1e3 1e3 1e3]  NominalFrequency=60  UnbalancedPower=off  ActivePower=0  InductivePower=0  CapacitivePower=1e-06  Pabc=[10e3 9e3 11e3]  QLabc=[100 90 110]  QCabc=[100 90 110]  Pabcp=[10e3 9e3 11e3]  QLabcp=[100 90 110]  QCabcp=[100 90 110]  Measurements=None  LoadType=constant PQ
  VI Recorder8 : Subsystem
  InPhaseA : PMIOPort  Side=Left
  InPhaseB : PMIOPort  Port=2  Side=Left
  InPhaseC : PMIOPort  Port=3  Side=Left
  OutPhaseA : PMIOPort  Port=4  Side=Right
  OutPhaseB : PMIOPort  Port=5  Side=Right
  OutPhaseC : PMIOPort  Port=6  Side=Right
  wires:
  Bus_5/2 -> VI Recorder8/2(Irec)
  Bus_5/1 -> VI Recorder8/1(Vrec)
  connections:
  Bus Load 5/LConn1 -- OutPhaseA/RConn1 -- Capacitor 5/LConn1 -- Bus_5/RConn1
  Bus_5/RConn2 -- OutPhaseB/RConn1 -- Capacitor 5/LConn2 -- Bus Load 5/LConn2
  Bus_5/RConn3 -- OutPhaseC/RConn1 -- Capacitor 5/LConn3 -- Bus Load 5/LConn3
  InPhaseA/RConn1 -- Bus_5/LConn1
  InPhaseB/RConn1 -- Bus_5/LConn2
  InPhaseC/RConn1 -- Bus_5/LConn3

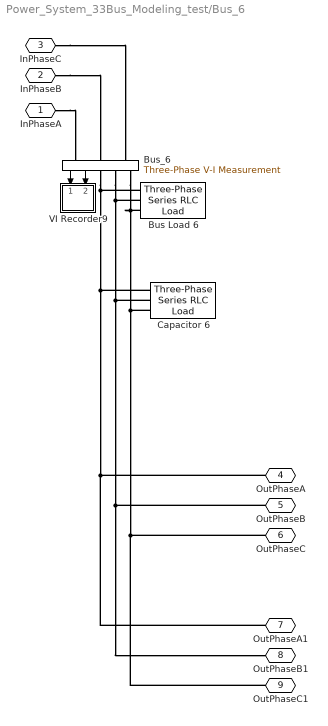
== system Power_System_33Bus_Modeling_test/Bus_6 ==
  Bus Load 6 : spsThreePhaseSeriesRLCLoadLib/Three-Phase Series RLC Load  LConnTagsString=A|B|C  Configuration=Y (grounded)  NominalVoltage=22900  Vabc=[1e3 1e3 1e3]  Vabcp=[1e3 1e3 1e3]  NominalFrequency=60  UnbalancedPower=off  ActivePower=300e3  InductivePower=100e3  CapacitivePower=0  Pabc=[10e3 9e3 11e3]  QLabc=[100 90 110]  QCabc=[100 90 110]  Pabcp=[10e3 9e3 11e3]  QLabcp=[100 90 110]  QCabcp=[100 90 110]  Measurements=None  LoadType=constant PQ
  Bus_6 : spsThreePhaseVIMeasurementLib/Three-Phase V-I Measurement  VoltageMeasurement=phase-to-phase  SetLabelV=off  LabelV=Vabc  Vpu=off  VpuLL=off  CurrentMeasurement=yes  SetLabelI=off  LabelI=Iabc  Ipu=off  Pbase=100e6  Vbase=500e3  OutputType=Complex  PhasorSimulation=off  PSBequivalent=0
  Capacitor 6 : spsThreePhaseSeriesRLCLoadLib/Three-Phase Series RLC Load  LConnTagsString=A|B|C  Configuration=Y (grounded)  NominalVoltage=22900  Vabc=[1e3 1e3 1e3]  Vabcp=[1e3 1e3 1e3]  NominalFrequency=60  UnbalancedPower=off  ActivePower=0  InductivePower=0  CapacitivePower=1e-06  Pabc=[10e3 9e3 11e3]  QLabc=[100 90 110]  QCabc=[100 90 110]  Pabcp=[10e3 9e3 11e3]  QLabcp=[100 90 110]  QCabcp=[100 90 110]  Measurements=None  LoadType=constant PQ
  VI Recorder9 : Subsystem
  InPhaseA : PMIOPort  Side=Left
  InPhaseB : PMIOPort  Port=2  Side=Left
  InPhaseC : PMIOPort  Port=3  Side=Left
  OutPhaseA : PMIOPort  Port=4  Side=Right
  OutPhaseB : PMIOPort  Port=5  Side=Right
  OutPhaseC : PMIOPort  Port=6  Side=Right
  OutPhaseA1 : PMIOPort  Port=7  Side=Right
  OutPhaseB1 : PMIOPort  Port=8  Side=Right
  OutPhaseC1 : PMIOPort  Port=9  Side=Right
  wires:
  Bus_6/1 -> VI Recorder9/1(Vrec)
  Bus_6/2 -> VI Recorder9/2(Irec)
  connections:
  Bus Load 6/LConn1 -- Capacitor 6/LConn1 -- OutPhaseA1/RConn1 -- OutPhaseA/RConn1 -- Bus_6/RConn1
  Bus Load 6/LConn3 -- Capacitor 6/LConn3 -- OutPhaseC1/RConn1 -- OutPhaseC/RConn1 -- Bus_6/RConn3
  Bus Load 6/LConn2 -- Capacitor 6/LConn2 -- OutPhaseB/RConn1 -- OutPhaseB1/RConn1 -- Bus_6/RConn2
  InPhaseA/RConn1 -- Bus_6/LConn1
  InPhaseB/RConn1 -- Bus_6/LConn2
  InPhaseC/RConn1 -- Bus_6/LConn3

== system Power_System_33Bus_Modeling_test/Bus_7 ==
  Bus Load 7 : spsThreePhaseSeriesRLCLoadLib/Three-Phase Series RLC Load  LConnTagsString=A|B|C  Configuration=Y (grounded)  NominalVoltage=22900  Vabc=[1e3 1e3 1e3]  Vabcp=[1e3 1e3 1e3]  NominalFrequency=60  UnbalancedPower=off  ActivePower=1000e3  InductivePower=500e3  CapacitivePower=0  Pabc=[10e3 9e3 11e3]  QLabc=[100 90 110]  QCabc=[100 90 110]  Pabcp=[10e3 9e3 11e3]  QLabcp=[100 90 110]  QCabcp=[100 90 110]  Measurements=None  LoadType=constant PQ
  Bus_7 : spsThreePhaseVIMeasurementLib/Three-Phase V-I Measurement  VoltageMeasurement=phase-to-phase  SetLabelV=off  LabelV=Vabc  Vpu=off  VpuLL=off  CurrentMeasurement=yes  SetLabelI=off  LabelI=Iabc  Ipu=off  Pbase=100e6  Vbase=500e3  OutputType=Complex  PhasorSimulation=off  PSBequivalent=0
  Capacitor 7 : spsThreePhaseSeriesRLCLoadLib/Three-Phase Series RLC Load  LConnTagsString=A|B|C  Configuration=Y (grounded)  NominalVoltage=22900  Vabc=[1e3 1e3 1e3]  Vabcp=[1e3 1e3 1e3]  NominalFrequency=60  UnbalancedPower=off  ActivePower=0  InductivePower=0  CapacitivePower=1e-06  Pabc=[10e3 9e3 11e3]  QLabc=[100 90 110]  QCabc=[100 90 110]  Pabcp=[10e3 9e3 11e3]  QLabcp=[100 90 110]  QCabcp=[100 90 110]  Measurements=None  LoadType=constant PQ
  VI Recorder10 : Subsystem
  InPhaseA : PMIOPort  Side=Left
  InPhaseB : PMIOPort  Port=2  Side=Left
  InPhaseC : PMIOPort  Port=3  Side=Left
  OutPhaseA : PMIOPort  Port=4  Side=Right
  OutPhaseB : PMIOPort  Port=5  Side=Right
  OutPhaseC : PMIOPort  Port=6  Side=Right
  wires:
  Bus_7/2 -> VI Recorder10/2(Irec)
  Bus_7/1 -> VI Recorder10/1(Vrec)
  connections:
  Bus_7/RConn1 -- OutPhaseA/RConn1 -- Capacitor 7/LConn1 -- Bus Load 7/LConn1
  Bus Load 7/LConn2 -- OutPhaseB/RConn1 -- Capacitor 7/LConn2 -- Bus_7/RConn2
  Capacitor 7/LConn3 -- OutPhaseC/RConn1 -- Bus Load 7/LConn3 -- Bus_7/RConn3
  InPhaseA/RConn1 -- Bus_7/LConn1
  InPhaseB/RConn1 -- Bus_7/LConn2
  InPhaseC/RConn1 -- Bus_7/LConn3

== system Power_System_33Bus_Modeling_test/Bus_8 ==
  Bus Load 8 : spsThreePhaseSeriesRLCLoadLib/Three-Phase Series RLC Load  LConnTagsString=A|B|C  Configuration=Y (grounded)  NominalVoltage=22900  Vabc=[1e3 1e3 1e3]  Vabcp=[1e3 1e3 1e3]  NominalFrequency=60  UnbalancedPower=off  ActivePower=1000e3  InductivePower=500e3  CapacitivePower=0  Pabc=[10e3 9e3 11e3]  QLabc=[100 90 110]  QCabc=[100 90 110]  Pabcp=[10e3 9e3 11e3]  QLabcp=[100 90 110]  QCabcp=[100 90 110]  Measurements=None  LoadType=constant PQ
  Bus_8 : spsThreePhaseVIMeasurementLib/Three-Phase V-I Measurement  VoltageMeasurement=phase-to-phase  SetLabelV=off  LabelV=Vabc  Vpu=off  VpuLL=off  CurrentMeasurement=yes  SetLabelI=off  LabelI=Iabc  Ipu=off  Pbase=100e6  Vbase=500e3  OutputType=Complex  PhasorSimulation=off  PSBequivalent=0
  Capacitor 8 : spsThreePhaseSeriesRLCLoadLib/Three-Phase Series RLC Load  LConnTagsString=A|B|C  Configuration=Y (grounded)  NominalVoltage=22900  Vabc=[1e3 1e3 1e3]  Vabcp=[1e3 1e3 1e3]  NominalFrequency=60  UnbalancedPower=off  ActivePower=0  InductivePower=0  CapacitivePower=1e-06  Pabc=[10e3 9e3 11e3]  QLabc=[100 90 110]  QCabc=[100 90 110]  Pabcp=[10e3 9e3 11e3]  QLabcp=[100 90 110]  QCabcp=[100 90 110]  Measurements=None  LoadType=constant PQ
  VI Recorder11 : Subsystem
  OutPhaseA : PMIOPort  Side=Right
  OutPhaseB : PMIOPort  Port=2  Side=Right
  OutPhaseC : PMIOPort  Port=3  Side=Right
  InPhaseA1 : PMIOPort  Port=4  Side=Left
  InPhaseB1 : PMIOPort  Port=5  Side=Left
  InPhaseC1 : PMIOPort  Port=6  Side=Left
  wires:
  Bus_8/2 -> VI Recorder11/2(Irec)
  Bus_8/1 -> VI Recorder11/1(Vrec)
  connections:
  Bus Load 8/LConn1 -- OutPhaseA/RConn1 -- Capacitor 8/LConn1 -- Bus_8/RConn1
  Bus Load 8/LConn2 -- OutPhaseB/RConn1 -- Capacitor 8/LConn2 -- Bus_8/RConn2
  Bus_8/RConn3 -- OutPhaseC/RConn1 -- Capacitor 8/LConn3 -- Bus Load 8/LConn3
  InPhaseA1/RConn1 -- Bus_8/LConn1
  InPhaseB1/RConn1 -- Bus_8/LConn2
  InPhaseC1/RConn1 -- Bus_8/LConn3

== system Power_System_33Bus_Modeling_test/Bus_9 ==
  Bus Load 9 : spsThreePhaseSeriesRLCLoadLib/Three-Phase Series RLC Load  LConnTagsString=A|B|C  Configuration=Y (grounded)  NominalVoltage=22900  Vabc=[1e3 1e3 1e3]  Vabcp=[1e3 1e3 1e3]  NominalFrequency=60  UnbalancedPower=off  ActivePower=300e3  InductivePower=100e3  CapacitivePower=0  Pabc=[10e3 9e3 11e3]  QLabc=[100 90 110]  QCabc=[100 90 110]  Pabcp=[10e3 9e3 11e3]  QLabcp=[100 90 110]  QCabcp=[100 90 110]  Measurements=None  LoadType=constant PQ
  Bus_9 : spsThreePhaseVIMeasurementLib/Three-Phase V-I Measurement  VoltageMeasurement=phase-to-phase  SetLabelV=off  LabelV=Vabc  Vpu=off  VpuLL=off  CurrentMeasurement=yes  SetLabelI=off  LabelI=Iabc  Ipu=off  Pbase=100e6  Vbase=500e3  OutputType=Complex  PhasorSimulation=off  PSBequivalent=0
  Capacitor 9 : spsThreePhaseSeriesRLCLoadLib/Three-Phase Series RLC Load  LConnTagsString=A|B|C  Configuration=Y (grounded)  NominalVoltage=22900  Vabc=[1e3 1e3 1e3]  Vabcp=[1e3 1e3 1e3]  NominalFrequency=60  UnbalancedPower=off  ActivePower=0  InductivePower=0  CapacitivePower=1e-06  Pabc=[10e3 9e3 11e3]  QLabc=[100 90 110]  QCabc=[100 90 110]  Pabcp=[10e3 9e3 11e3]  QLabcp=[100 90 110]  QCabcp=[100 90 110]  Measurements=None  LoadType=constant PQ
  VI Recorder12 : Subsystem
  InPhaseA : PMIOPort  Side=Left
  InPhaseB : PMIOPort  Port=2  Side=Left
  InPhaseC : PMIOPort  Port=3  Side=Left
  OutPhaseA : PMIOPort  Port=4  Side=Right
  OutPhaseB : PMIOPort  Port=5  Side=Right
  OutPhaseC : PMIOPort  Port=6  Side=Right
  wires:
  Bus_9/2 -> VI Recorder12/2(Irec)
  Bus_9/1 -> VI Recorder12/1(Vrec)
  connections:
  Capacitor 9/LConn1 -- OutPhaseA/RConn1 -- Bus Load 9/LConn1 -- Bus_9/RConn1
  Capacitor 9/LConn2 -- OutPhaseB/RConn1 -- Bus_9/RConn2 -- Bus Load 9/LConn2
  Bus Load 9/LConn3 -- Bus_9/RConn3 -- OutPhaseC/RConn1 -- Capacitor 9/LConn3
  InPhaseA/RConn1 -- Bus_9/LConn1
  InPhaseB/RConn1 -- Bus_9/LConn2
  InPhaseC/RConn1 -- Bus_9/LConn3

== system Power_System_33Bus_Modeling_test/Bus_10/VI Recorder13 ==
  Vrec : Inport
  Irec : Inport  Port=2
  tag scope: I9to10=global, V9to10=global
  wires:
  Vrec/1 -> [V9to10]
  Irec/1 -> [I9to10]

== system Power_System_33Bus_Modeling_test/Bus_11/VI Recorder14 ==
  Vrec : Inport
  Irec : Inport  Port=2
  tag scope: I10to11=global, V10to11=global
  wires:
  Vrec/1 -> [V10to11]
  Irec/1 -> [I10to11]

== system Power_System_33Bus_Modeling_test/Bus_12/VI Recorder15 ==
  Vrec : Inport
  Irec : Inport  Port=2
  tag scope: I11to12=global, V11to12=global
  wires:
  Vrec/1 -> [V11to12]
  Irec/1 -> [I11to12]

== system Power_System_33Bus_Modeling_test/Bus_13/VI Recorder16 ==
  Vrec : Inport
  Irec : Inport  Port=2
  tag scope: I12to13=global, V12to13=global
  wires:
  Vrec/1 -> [V12to13]
  Irec/1 -> [I12to13]

== system Power_System_33Bus_Modeling_test/Bus_14/VI Recorder17 ==
  Vrec : Inport
  Irec : Inport  Port=2
  tag scope: I13to14=global, V13to14=global
  wires:
  Vrec/1 -> [V13to14]
  Irec/1 -> [I13to14]

== system Power_System_33Bus_Modeling_test/Bus_15/VI Recorder18 ==
  Vrec : Inport
  Irec : Inport  Port=2
  tag scope: I14to15=global, V14to15=global
  wires:
  Vrec/1 -> [V14to15]
  Irec/1 -> [I14to15]

== system Power_System_33Bus_Modeling_test/Bus_16/VI Recorder19 ==
  Vrec : Inport
  Irec : Inport  Port=2
  tag scope: I15to16=global, V15to16=global
  wires:
  Vrec/1 -> [V15to16]
  Irec/1 -> [I15to16]

== system Power_System_33Bus_Modeling_test/Bus_17/VI Recorder20 ==
  Vrec : Inport
  Irec : Inport  Port=2
  tag scope: I16to17=global, V16to17=global
  wires:
  Vrec/1 -> [V16to17]
  Irec/1 -> [I16to17]

== system Power_System_33Bus_Modeling_test/Bus_18/VI Recorder21 ==
  Vrec : Inport
  Irec : Inport  Port=2
  tag scope: I17to18=global, V17to18=global
  wires:
  Vrec/1 -> [V17to18]
  Irec/1 -> [I17to18]

== system Power_System_33Bus_Modeling_test/Bus_19/VI Recorder ==
  Vrec : Inport
  Irec : Inport  Port=2
  tag scope: I2to19=global, V2to19=global
  wires:
  Vrec/1 -> [V2to19]
  Irec/1 -> [I2to19]

== system Power_System_33Bus_Modeling_test/Bus_2/VI Recorder5 ==
  Vrec : Inport
  Irec : Inport  Port=2
  tag scope: I1to2=global, V1to2=global
  wires:
  Vrec/1 -> [V1to2]
  Irec/1 -> [I1to2]

== system Power_System_33Bus_Modeling_test/Bus_20/VI Recorder1 ==
  Vrec : Inport
  Irec : Inport  Port=2
  tag scope: I19to20=global, V19to20=global
  wires:
  Vrec/1 -> [V19to20]
  Irec/1 -> [I19to20]

== system Power_System_33Bus_Modeling_test/Bus_21/VI Recorder2 ==
  Vrec : Inport
  Irec : Inport  Port=2
  tag scope: I20to21=global, V20to21=global
  wires:
  Vrec/1 -> [V20to21]
  Irec/1 -> [I20to21]

== system Power_System_33Bus_Modeling_test/Bus_22/VI Recorder3 ==
  Vrec : Inport
  Irec : Inport  Port=2
  tag scope: I21to22=global, V21to22=global
  wires:
  Vrec/1 -> [V21to22]
  Irec/1 -> [I21to22]

== system Power_System_33Bus_Modeling_test/Bus_23/VI Recorder32 ==
  Vrec : Inport
  Irec : Inport  Port=2
  tag scope: I3to23=global, V3to23=global
  wires:
  Vrec/1 -> [V3to23]
  Irec/1 -> [I3to23]

== system Power_System_33Bus_Modeling_test/Bus_24/VI Recorder31 ==
  Vrec : Inport
  Irec : Inport  Port=2
  tag scope: I23to24=global, V23to24=global
  wires:
  Vrec/1 -> [V23to24]
  Irec/1 -> [I23to24]

== system Power_System_33Bus_Modeling_test/Bus_25/VI Recorder30 ==
  Vrec : Inport
  Irec : Inport  Port=2
  tag scope: I24to25=global, V24to25=global
  wires:
  Vrec/1 -> [V24to25]
  Irec/1 -> [I24to25]

== system Power_System_33Bus_Modeling_test/Bus_26/VI Recorder22 ==
  Vrec : Inport
  Irec : Inport  Port=2
  tag scope: I6to26=global, V6to26=global
  wires:
  Vrec/1 -> [V6to26]
  Irec/1 -> [I6to26]

== system Power_System_33Bus_Modeling_test/Bus_27/VI Recorder23 ==
  Vrec : Inport
  Irec : Inport  Port=2
  tag scope: I26to27=global, V26to27=global
  wires:
  Vrec/1 -> [V26to27]
  Irec/1 -> [I26to27]

== system Power_System_33Bus_Modeling_test/Bus_28/VI Recorder24 ==
  Vrec : Inport
  Irec : Inport  Port=2
  tag scope: I27to28=global, V27to28=global
  wires:
  Vrec/1 -> [V27to28]
  Irec/1 -> [I27to28]

== system Power_System_33Bus_Modeling_test/Bus_29/VI Recorder25 ==
  Vrec : Inport
  Irec : Inport  Port=2
  tag scope: I28to29=global, V28to29=global
  wires:
  Vrec/1 -> [V28to29]
  Irec/1 -> [I28to29]

== system Power_System_33Bus_Modeling_test/Bus_3/VI Recorder6 ==
  Vrec : Inport
  Irec : Inport  Port=2
  tag scope: I2to3=global, V2to3=global
  wires:
  Vrec/1 -> [V2to3]
  Irec/1 -> [I2to3]

== system Power_System_33Bus_Modeling_test/Bus_30/VI Recorder26 ==
  Vrec : Inport
  Irec : Inport  Port=2
  tag scope: I29to30=global, V29to30=global
  wires:
  Vrec/1 -> [V29to30]
  Irec/1 -> [I29to30]

== system Power_System_33Bus_Modeling_test/Bus_31/VI Recorder27 ==
  Vrec : Inport
  Irec : Inport  Port=2
  tag scope: I30to31=global, V30to31=global
  wires:
  Vrec/1 -> [V30to31]
  Irec/1 -> [I30to31]

== system Power_System_33Bus_Modeling_test/Bus_32/VI Recorder28 ==
  Vrec : Inport
  Irec : Inport  Port=2
  tag scope: I31to32=global, V31to32=global
  wires:
  Vrec/1 -> [V31to32]
  Irec/1 -> [I31to32]

== system Power_System_33Bus_Modeling_test/Bus_33/VI Recorder29 ==
  Vrec : Inport
  Irec : Inport  Port=2
  tag scope: I32to33=global, V32to33=global
  wires:
  Vrec/1 -> [V32to33]
  Irec/1 -> [I32to33]

== system Power_System_33Bus_Modeling_test/Bus_4/VI Recorder7 ==
  Vrec : Inport
  Irec : Inport  Port=2
  tag scope: I3to4=global, V3to4=global
  wires:
  Vrec/1 -> [V3to4]
  Irec/1 -> [I3to4]

== system Power_System_33Bus_Modeling_test/Bus_5/VI Recorder8 ==
  Vrec : Inport
  Irec : Inport  Port=2
  tag scope: I4to5=global, V4to5=global
  wires:
  Vrec/1 -> [V4to5]
  Irec/1 -> [I4to5]

== system Power_System_33Bus_Modeling_test/Bus_6/VI Recorder9 ==
  Vrec : Inport
  Irec : Inport  Port=2
  tag scope: I5to6=global, V5to6=global
  wires:
  Vrec/1 -> [V5to6]
  Irec/1 -> [I5to6]

== system Power_System_33Bus_Modeling_test/Bus_7/VI Recorder10 ==
  Vrec : Inport
  Irec : Inport  Port=2
  tag scope: I6to7=global, V6to7=global
  wires:
  Vrec/1 -> [V6to7]
  Irec/1 -> [I6to7]

== system Power_System_33Bus_Modeling_test/Bus_8/VI Recorder11 ==
  Vrec : Inport
  Irec : Inport  Port=2
  tag scope: I7to8=global, V7to8=global
  wires:
  Vrec/1 -> [V7to8]
  Irec/1 -> [I7to8]

== system Power_System_33Bus_Modeling_test/Bus_9/VI Recorder12 ==
  Vrec : Inport
  Irec : Inport  Port=2
  tag scope: I8to9=global, V8to9=global
  wires:
  Vrec/1 -> [V8to9]
  Irec/1 -> [I8to9]
